simulink model "m006_Bucket"  (R2022a)
settings: Solver=VariableStepAuto  StartTime=0.0  StopTime=10.0  RelTol=1e-3
settings Model: Creator=Admin  LastModifiedBy=Admin

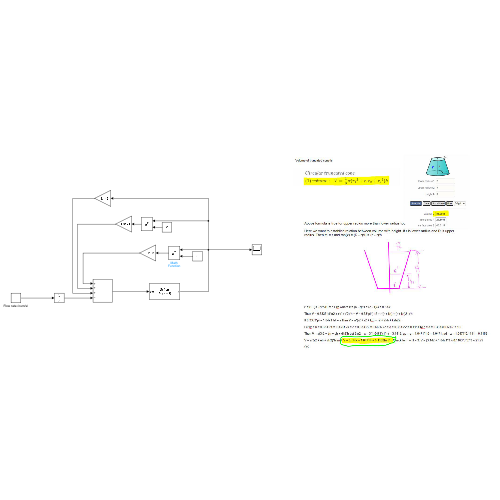
[thumbnail: Simulink's stored preview of the top-level diagram]
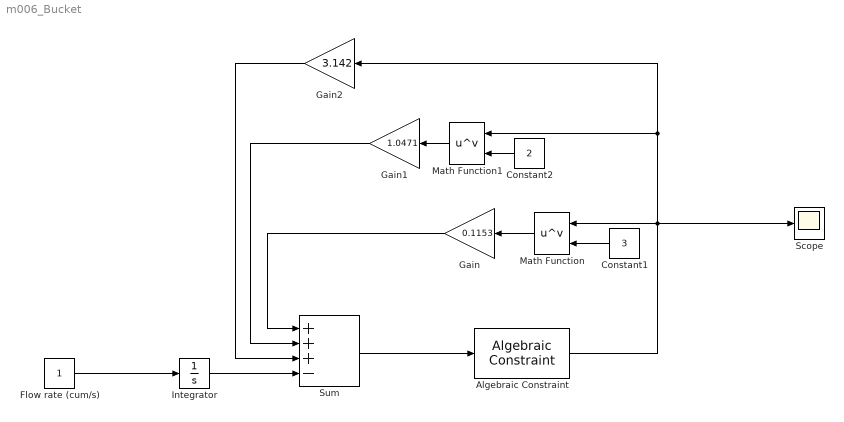
== system m006_Bucket ==
  Algebraic Constraint : AlgebraicConstraint
  Constant1 : Constant  Value=3
  Constant2 : Constant  Value=2
  Flow rate (cum/s) : Constant
  Gain : Gain  Gain=0.1153
  Gain1 : Gain  Gain=1.0471
  Gain2 : Gain  Gain=3.142
  Integrator : Integrator
  Math Function : Math  Operator=pow
  Math Function1 : Math  Operator=pow
  Scope : Scope
  Sum : Sum  Inputs=+++-
  wires:
  Constant1/1 -> Math Function/2
  Math Function/1 -> Gain/1
  Math Function1/1 -> Gain1/1
  Constant2/1 -> Math Function1/2
  Algebraic Constraint/1 -> Scope/1, Gain2/1, Math Function1/1, Math Function/1
  Gain2/1 -> Sum/3
  Gain1/1 -> Sum/2
  Gain/1 -> Sum/1
  Integrator/1 -> Sum/4
  Sum/1 -> Algebraic Constraint/1
  Flow rate (cum/s)/1 -> Integrator/1
